simulink model "model3"  (Simulink 5.0)
settings: Solver=ode4  SolverMode=SingleTasking  StartTime=0.0  StopTime=10.0  FixedStep=1e-2  RelTol=1e-3
values from neighbouring files (symbols this model uses):
  A = [0,0;0,-1]    [skrypt3.m]
  Aplus = expm(h * A)    [skrypt3.m]
  B = [1;1]    [skrypt3.m]
  Bplus = double( int( expm( s*A )*B, s, 0, h ) )    [skrypt3.m]
  C = eye(2)    [skrypt3.m]
  Cplus = C    [skrypt3.m]
  h = 0.1    [skrypt3.m]
settings Model: LastModifiedBy=Krzysiek  LimitDataPoints=off  RTWOptions="-aEnforceIntegerDowncast=1 -aExtMode=0 -aExtModeTesting=0 -aFoldNonRolledExpr=1 -aForceParamTrailComments=0 -aGenerateComments=1 -aGenerateReport=0 -aIgnoreCustomStorageClasses=1 -aIncDataTypeInIds=0 -aIncHierarchyInIds=0 -aInlineInvariantSignals=0 -aInlinedPrmAccess=\"Literals\" -aLocalBlockOutputs=1 -aLogVarNameModifier=\"rt_\" -aMaxRTWIdLen=31 -aPrefixModelToSubsysFcnNames=1 -aRTWVerbose=1 -aRollThreshold=5 -aShowEliminatedStatements=0"

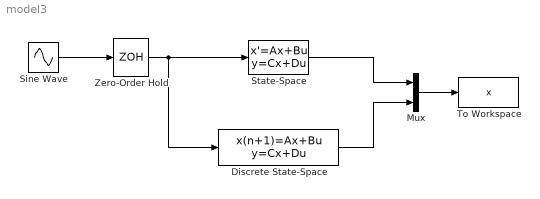
== system model3 ==
  Discrete State-Space : DiscreteStateSpace  A=Aplus  B=Bplus  C=Cplus  D=[0;0]  SampleTime=h
  Mux : Mux  Inputs=2
  Sine Wave : Sin  SampleTime=0
  State-Space : StateSpace  A=A  B=B  C=C  D=[0;0]
  To Workspace : ToWorkspace  VariableName=x  SampleTime=-1  SaveFormat=Array
  Zero-Order Hold : ZeroOrderHold  SampleTime=h
  wires:
  Sine Wave/1 -> Zero-Order Hold/1
  Zero-Order Hold/1 -> State-Space/1, Discrete State-Space/1
  State-Space/1 -> Mux/1
  Discrete State-Space/1 -> Mux/2
  Mux/1 -> To Workspace/1
